simulink model "linear_test"  (R2020b)
settings: Solver=VariableStepAuto  StartTime=0.0  StopTime=1000.0  RelTol=1e-3
settings Model: Creator=BearHsia  LastModifiedBy=BearHsia

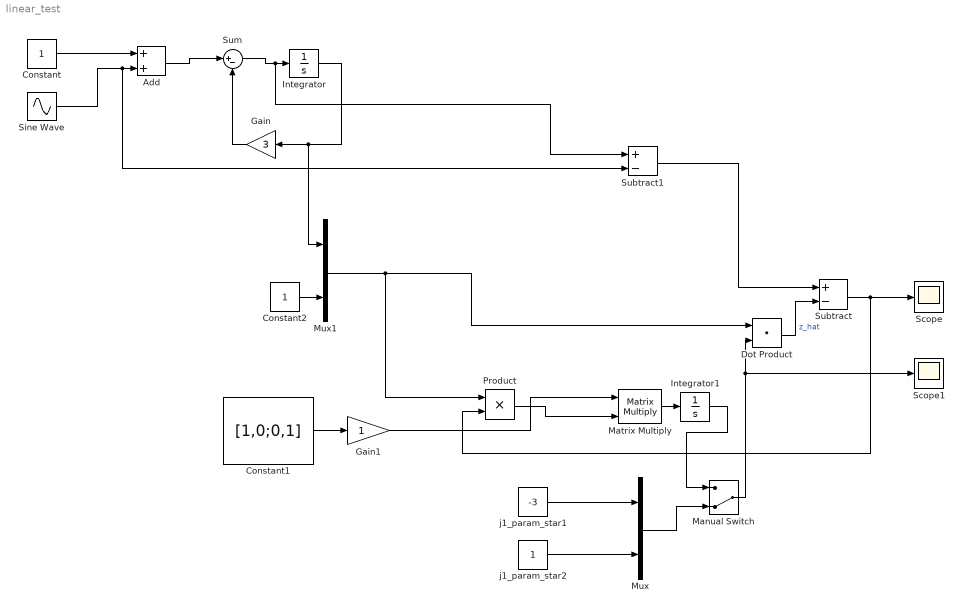
== system linear_test ==
  Add : Sum
  Constant : Constant
  Constant1 : Constant  Value=[1,0;0,1]
  Constant2 : Constant
  Dot Product : DotProduct  InputSameDT=on  OutDataTypeStr=Inherit: Inherit via internal rule
  Gain : Gain  Gain=3
  Gain1 : Gain
  Integrator : Integrator
  Integrator1 : Integrator  InitialCondition=[0;0]
  Manual Switch : ManualSwitch  CurrentSetting=0
  Matrix Multiply : Product  Multiplication=Matrix(*)
  Mux : Mux  Inputs=2
  Mux1 : Mux  Inputs=2
  Product : Product
  Scope : Scope
  Scope1 : Scope
  Sine Wave : Sin  Frequency=2  SampleTime=0
  Subtract : Sum  Inputs=+-
  Subtract1 : Sum  Inputs=+-
  Sum : Sum  Inputs=|+-
  j1_param_star1 : Constant  Value=-3
  j1_param_star2 : Constant
  wires:
  Integrator/1 -> Mux1/1, Gain/1
  Gain/1 -> Sum/2
  Sum/1 -> Subtract1/1, Integrator/1
  Add/1 -> Sum/1
  Mux/1 -> Manual Switch/2
  Matrix Multiply/1 -> Integrator1/1
  Mux1/1 -> Dot Product/1, Product/1
  j1_param_star2/1 -> Mux/2
  Manual Switch/1 -> Scope1/1, Dot Product/2
  Dot Product/1 -> Subtract/2  "z_hat"
  Constant1/1 -> Gain1/1
  Integrator1/1 -> Manual Switch/1
  Product/1 -> Matrix Multiply/2
  Gain1/1 -> Matrix Multiply/1
  Subtract/1 -> Scope/1, Product/2
  j1_param_star1/1 -> Mux/1
  Sine Wave/1 -> Subtract1/2, Add/2
  Constant/1 -> Add/1
  Subtract1/1 -> Subtract/1
  Constant2/1 -> Mux1/2
